simulink model "simulazione_004_s"  (R2016b)
settings: Solver=ode4  StartTime=0.0  StopTime=t_sim  FixedStep=step  RelTol=1e-3
values from neighbouring files (symbols this model uses):
  final_theta = 3*pi/2    (= 4.71238898038)    [simulazione_004_init.m]
  gain = 30 * eye(6)    [simulazione_004_init.m]
  motion_time = 5    [simulazione_004_init.m]
  movement_lower_limit = -movement_upper_limit    [simulazione_004_init.m]
  movement_upper_limit = [2*pi; 2*pi; 2*pi; 2*pi; 2*pi; 2*pi]    [simulazione_004_init.m]
  p_init = direct_kinematic(q_init)    [simulazione_004_init.m]
  q_init = [pi/2; -pi/3; -pi/9; pi/6; -pi/6; 0]    [simulazione_004_init.m]
  radius = 0.4    [simulazione_004_init.m]
  velocity_lower_limit = -velocity_upper_limit    [simulazione_004_init.m]
  velocity_upper_limit = [2*pi/3; 2*pi/3; pi; pi; pi; pi]    [simulazione_004_init.m]
settings Model: Creator=IBM  LastModifiedBy=IBM

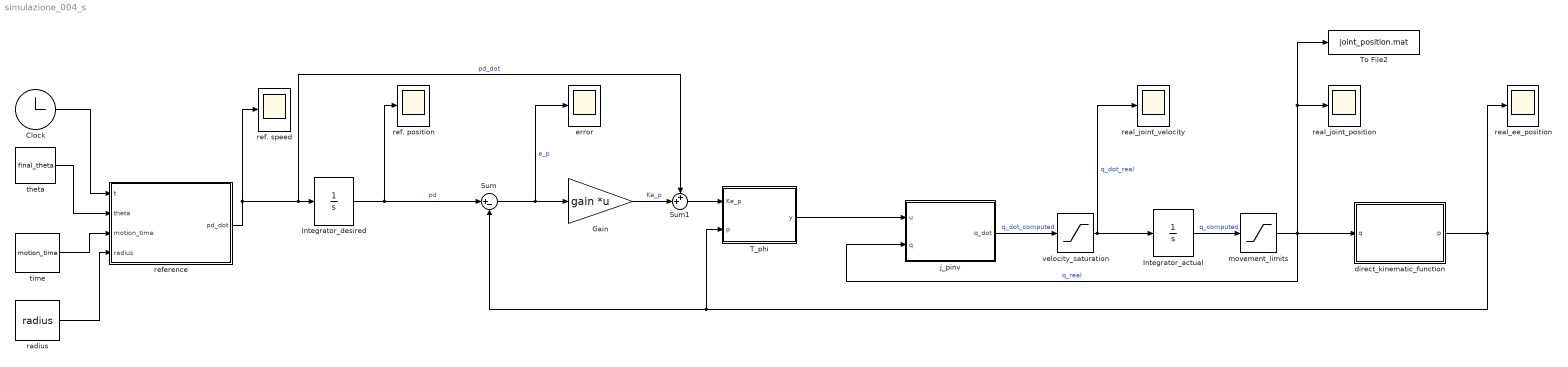
== system simulazione_004_s ==
  Clock : Clock
  Gain : Gain  Gain=gain  Multiplication=Matrix(K*u) (u vector)
  Integrator_actual : Integrator  InitialCondition=q_init
  Integrator_desired : Integrator  InitialCondition=p_init
  Sum : Sum  Inputs=|+-
  Sum1 : Sum  Inputs=++|
  T_phi : MATLAB Function  TreatAsAtomicUnit=on
  To File2 : ToFile  Filename=joint_position.mat  MatrixName=q
  direct_kinematic_function : MATLAB Function  TreatAsAtomicUnit=on
  error : Scope
  j_pinv : MATLAB Function  TreatAsAtomicUnit=on
  movement_limits : Saturate  UpperLimit=movement_upper_limit  LowerLimit=movement_lower_limit
  radius : Constant  Value=radius
  real_ee_position : Scope
  real_joint_position : Scope
  real_joint_velocity : Scope
  ref. position : Scope
  ref. speed : Scope
  reference : MATLAB Function  TreatAsAtomicUnit=on
  theta : Constant  Value=final_theta
  time : Constant  Value=motion_time
  velocity_saturation : Saturate  UpperLimit=velocity_upper_limit  LowerLimit=velocity_lower_limit
  wires:
  Clock/1 -> reference/1(t)
  Integrator_desired/1 -> ref. position/1, Sum/1  "pd"
  Sum/1 -> error/1, Gain/1  "e_p"
  direct_kinematic_function/1(p) -> real_ee_position/1, T_phi/2(p), Sum/2
  theta/1 -> reference/2(theta)
  reference/1(pd_dot) -> ref. speed/1, Sum1/1, Integrator_desired/1  "pd_dot"
  time/1 -> reference/3(motion_time)
  radius/1 -> reference/4(radius)
  Integrator_actual/1 -> movement_limits/1  "q_computed"
  movement_limits/1 -> j_pinv/2(q), To File2/1, real_joint_position/1, direct_kinematic_function/1(q)  "q_real"
  j_pinv/1(q_dot) -> velocity_saturation/1  "q_dot_computed"
  velocity_saturation/1 -> real_joint_velocity/1, Integrator_actual/1  "q_dot_real"
  Gain/1 -> Sum1/2  "Ke_p"
  Sum1/1 -> T_phi/1(Ke_p)
  T_phi/1(y) -> j_pinv/1(u)

== matlab function simulazione_004_s/j_pinv ==
  data: u input; q_dot output; q input
function q_dot = j_pinv(u, q)
    
    J = geometric_jacobian(q);    
    J_p = pinv(J);
    q_dot = J_p*u;
    
end

== matlab function simulazione_004_s/reference ==
  data: t input; theta input; pd_dot output; motion_time input; radius input
function pd_dot = reference(t, theta, motion_time, radius)

    pd_dot = rotational_reference(t, theta, motion_time, radius);
    
end

== matlab function simulazione_004_s/direct_kinematic_function ==
  data: q input; p output
function p = dkf(q)

    p = direct_kinematic(q);

== matlab function simulazione_004_s/T_phi ==
  data: Ke_p input; y output; p input
function y = T_phi(Ke_p, p)
        
    t_phi_matrix = [0,  -sin(p(4)),     cos(p(4))*sin(p(5));
                    0,   cos(p(4)),     sin(p(4))*sin(p(5));
                    1,       0,             cos(p(5))];
            
    t_phi_matrix_6x6 = [ eye(3),   zeros(3);
                        zeros(3), t_phi_matrix];
    
    y = t_phi_matrix_6x6 * Ke_p;
end
